simulink model "B_ctrb"  (R2015a)
settings: Solver=ode45  StartTime=0.0  StopTime=50  RelTol=1e-3
values from neighbouring files (symbols this model uses):
  A1 = [-0.125 0 0;1 0 0;0 1 0]    [A_tftf.m]
  B1 = [1;0;0]    [A_tftf.m]
  C1 = [0 -0.0883 -0.0044]    [A_tftf.m]
  D1 = 0    [A_tftf.m]
  K = lqr(a,b,Q,R)    [A_tftf.m]
libraries: simulink x3
settings Model: Creator=HomeTown  LastModifiedBy=HomeTown

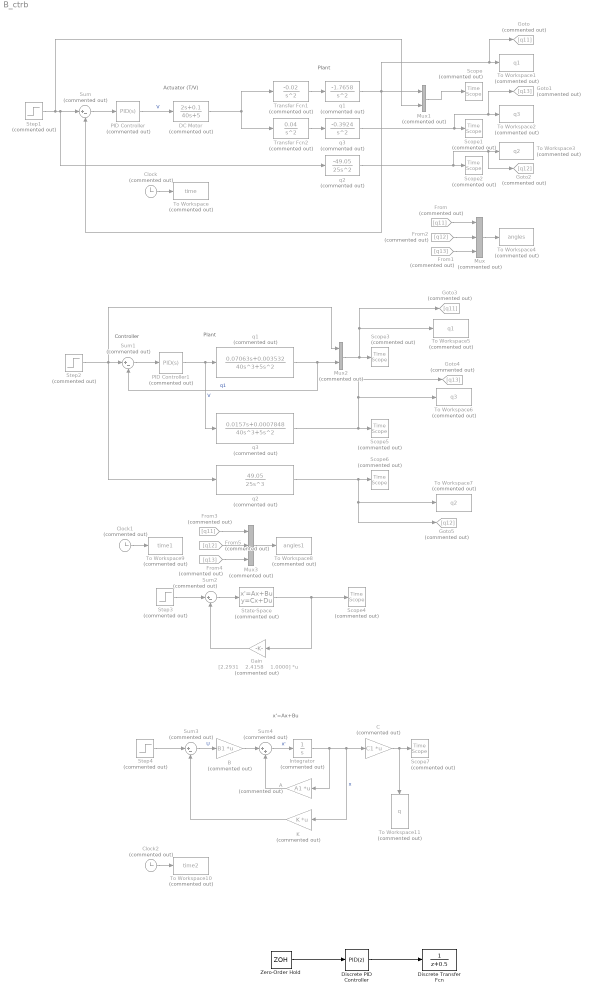
== system B_ctrb ==
  note: x'=Ax+Bu
  note: Controller
  note: Plant
  note: Plant
  note: Actuator (T/V)
  A : Gain  Commented=on  Gain=A1  Multiplication=Matrix(K*u)
  B : Gain  Commented=on  Gain=B1  Multiplication=Matrix(K*u)
  C : Gain  Commented=on  Gain=C1  Multiplication=Matrix(K*u)
  Clock : Clock  Commented=on
  Clock1 : Clock  Commented=on
  Clock2 : Clock  Commented=on
  DC Motor : TransferFcn  Commented=on  Numerator=[2 0.1]  Denominator=[40 5]
  Discrete Transfer Fcn : DiscreteTransferFcn
  Discrete PID Controller : simulink/Continuous/PID Controller  Controller=PID  TimeDomain=Discrete-time  SampleTime=1  IntegratorMethod=Forward Euler  FilterMethod=Forward Euler  Form=Parallel  UseFilter=on  ControllerParametersSource=internal  P=21.1  I=26  D=0  N=100  InitialConditionSource=internal  InitialConditionForIntegrator=0  InitialConditionForFilter=0  ExternalReset=none  LimitOutput=off  UpperSaturationLimit=inf  LowerSaturationLimit=-inf  LinearizeAsGain=off  AntiWindupMode=none  Kb=1  TrackingMode=off  Kt=1  PParamMin=[]  PParamMax=[]  IParamMin=[]  IParamMax=[]  DParamMin=[]  DParamMax=[]  NParamMin=[]  NParamMax=[]  KbParamMin=[]  KbParamMax=[]  KtParamMin=[]  KtParamMax=[]  POutMin=[]  POutMax=[]  IOutMin=[]  IOutMax=[]  DOutMin=[]  DOutMax=[]  NOutMin=[]  NOutMax=[]  KbOutMin=[]  KbOutMax=[]  KtOutMin=[]  KtOutMax=[]  IntegratorOutMin=[]  IntegratorOutMax=[]  FilterOutMin=[]  FilterOutMax=[]  SumOutMin=[]  SumOutMax=[]  SumI1OutMin=[]  SumI1OutMax=[]  SumI2OutMin=[]  SumI2OutMax=[]  SumI3OutMin=[]  SumI3OutMax=[]  SumDOutMin=[]  SumDOutMax=[]  SaturationOutMin=[]  SaturationOutMax=[]  IntegratorContinuousStateAttributes=''  IntegratorStateMustResolveToSignalObject=off  IntegratorRTWStateStorageClass=Auto  FilterContinuousStateAttributes=''  FilterStateMustResolveToSignalObject=off  FilterRTWStateStorageClass=Auto  DifferentiatorICPrevScaledInput=0  DifferentiatorOutMin=[]  DifferentiatorOutMax=[]
  From : From  Commented=on  GotoTag=q11
  From1 : From  Commented=on  GotoTag=q13
  From2 : From  Commented=on  GotoTag=q12
  From3 : From  Commented=on  GotoTag=q11
  From4 : From  Commented=on  GotoTag=q13
  From5 : From  Commented=on  GotoTag=q12
  Gain : Gain  Commented=on  Gain="[2.2931    2.4158    1.0000]"  Multiplication=Matrix(K*u)
  Goto : Goto  Commented=on  GotoTag=q11
  Goto1 : Goto  Commented=on  GotoTag=q13
  Goto2 : Goto  Commented=on  GotoTag=q12
  Goto3 : Goto  Commented=on  GotoTag=q11
  Goto4 : Goto  Commented=on  GotoTag=q13
  Goto5 : Goto  Commented=on  GotoTag=q12
  Integrator : Integrator  Commented=on
  K : Gain  Commented=on  Gain=K  Multiplication=Matrix(K*u)
  Mux : Mux  Commented=on  Inputs=3
  Mux1 : Mux  Commented=on  Inputs=2
  Mux2 : Mux  Commented=on  Inputs=2
  Mux3 : Mux  Commented=on  Inputs=3
  PID Controller : simulink/Continuous/PID Controller  Commented=on  Controller=PID  TimeDomain=Continuous-time  SampleTime=-1  IntegratorMethod=Forward Euler  FilterMethod=Forward Euler  Form=Parallel  UseFilter=on  ControllerParametersSource=internal  P=150000  I=11111  D=11  N=100  InitialConditionSource=internal  InitialConditionForIntegrator=0  InitialConditionForFilter=0  ExternalReset=none  LimitOutput=off  UpperSaturationLimit=inf  LowerSaturationLimit=-inf  LinearizeAsGain=on  AntiWindupMode=none  Kb=1  TrackingMode=off  Kt=1  PParamMin=[]  PParamMax=[]  IParamMin=[]  IParamMax=[]  DParamMin=[]  DParamMax=[]  NParamMin=[]  NParamMax=[]  KbParamMin=[]  KbParamMax=[]  KtParamMin=[]  KtParamMax=[]  POutMin=[]  POutMax=[]  IOutMin=[]  IOutMax=[]  DOutMin=[]  DOutMax=[]  NOutMin=[]  NOutMax=[]  KbOutMin=[]  KbOutMax=[]  KtOutMin=[]  KtOutMax=[]  IntegratorOutMin=[]  IntegratorOutMax=[]  FilterOutMin=[]  FilterOutMax=[]  SumOutMin=[]  SumOutMax=[]  SumI1OutMin=[]  SumI1OutMax=[]  SumI2OutMin=[]  SumI2OutMax=[]  SumI3OutMin=[]  SumI3OutMax=[]  SumDOutMin=[]  SumDOutMax=[]  SaturationOutMin=[]  SaturationOutMax=[]  IntegratorContinuousStateAttributes=''  IntegratorStateMustResolveToSignalObject=off  IntegratorRTWStateStorageClass=Auto  FilterContinuousStateAttributes=''  FilterStateMustResolveToSignalObject=off  FilterRTWStateStorageClass=Auto  DifferentiatorICPrevScaledInput=0  DifferentiatorOutMin=[]  DifferentiatorOutMax=[]
  PID Controller1 : simulink/Continuous/PID Controller  Commented=on  Controller=PID  TimeDomain=Continuous-time  SampleTime=-1  IntegratorMethod=Forward Euler  FilterMethod=Forward Euler  Form=Parallel  UseFilter=on  ControllerParametersSource=internal  P=350.723372354877  I=32.5997950441357  D=893.162577651587  N=8.93309035821885  InitialConditionSource=internal  InitialConditionForIntegrator=0  InitialConditionForFilter=0  ExternalReset=none  LimitOutput=off  UpperSaturationLimit=inf  LowerSaturationLimit=-inf  LinearizeAsGain=on  AntiWindupMode=none  Kb=1  TrackingMode=off  Kt=1  PParamMin=[]  PParamMax=[]  IParamMin=[]  IParamMax=[]  DParamMin=[]  DParamMax=[]  NParamMin=[]  NParamMax=[]  KbParamMin=[]  KbParamMax=[]  KtParamMin=[]  KtParamMax=[]  POutMin=[]  POutMax=[]  IOutMin=[]  IOutMax=[]  DOutMin=[]  DOutMax=[]  NOutMin=[]  NOutMax=[]  KbOutMin=[]  KbOutMax=[]  KtOutMin=[]  KtOutMax=[]  IntegratorOutMin=[]  IntegratorOutMax=[]  FilterOutMin=[]  FilterOutMax=[]  SumOutMin=[]  SumOutMax=[]  SumI1OutMin=[]  SumI1OutMax=[]  SumI2OutMin=[]  SumI2OutMax=[]  SumI3OutMin=[]  SumI3OutMax=[]  SumDOutMin=[]  SumDOutMax=[]  SaturationOutMin=[]  SaturationOutMax=[]  IntegratorContinuousStateAttributes=''  IntegratorStateMustResolveToSignalObject=off  IntegratorRTWStateStorageClass=Auto  FilterContinuousStateAttributes=''  FilterStateMustResolveToSignalObject=off  FilterRTWStateStorageClass=Auto  DifferentiatorICPrevScaledInput=0  DifferentiatorOutMin=[]  DifferentiatorOutMax=[]
  Scope{,1..7} (8 alike) : TimeScope  Commented=on
  State-Space : StateSpace  Commented=on  A=A1  B=B1  C=C1  D=D1  X0=0
  Step1 : Step  Commented=on  SampleTime=0
  Step2 : Step  Commented=on  SampleTime=0
  Step3 : Step  Commented=on  After=0  SampleTime=0
  Step4 : Step  Commented=on  SampleTime=0
  Sum{,1..3} (4 alike) : Sum  Commented=on  Inputs=|+-
  Sum4 : Sum  Commented=on  Inputs=|++
  To Workspace : ToWorkspace  Commented=on  VariableName=time  SampleTime=-1
  To Workspace1 : ToWorkspace  Commented=on  VariableName=q1  SampleTime=-1
  To Workspace10 : ToWorkspace  Commented=on  VariableName=time2  SampleTime=-1
  To Workspace11 : ToWorkspace  Commented=on  VariableName=q  SampleTime=-1
  To Workspace2 : ToWorkspace  Commented=on  VariableName=q3  SampleTime=-1
  To Workspace3 : ToWorkspace  Commented=on  VariableName=q2  SampleTime=-1
  To Workspace4 : ToWorkspace  Commented=on  VariableName=angles  SampleTime=-1
  To Workspace5 : ToWorkspace  Commented=on  VariableName=q1  SampleTime=-1
  To Workspace6 : ToWorkspace  Commented=on  VariableName=q3  SampleTime=-1
  To Workspace7 : ToWorkspace  Commented=on  VariableName=q2  SampleTime=-1
  To Workspace8 : ToWorkspace  Commented=on  VariableName=angles1  SampleTime=-1
  To Workspace9 : ToWorkspace  Commented=on  VariableName=time1  SampleTime=-1
  Transfer Fcn1 : TransferFcn  Commented=on  Numerator=[-0.02]  Denominator=[1 0 0]
  Transfer Fcn2 : TransferFcn  Commented=on  Numerator=[0.04]  Denominator=[1 0 0]
  Zero-Order Hold : ZeroOrderHold
  q1 : TransferFcn  Commented=on  Numerator=[-1.7658]  Denominator=[1 0 0]
  "q1  " : TransferFcn  Commented=on  Numerator=[0.07063 0.003532]  Denominator=[40 5 0 0]
  q2 : TransferFcn  Commented=on  Numerator=[-49.05]  Denominator=[25 0 0]
  "q2 " : TransferFcn  Commented=on  Numerator=[49.05]  Denominator=[25 0 0 0]
  q3 : TransferFcn  Commented=on  Numerator=[-0.3924]  Denominator=[1 0 0]
  "q3 " : TransferFcn  Commented=on  Numerator=[0.0157 0.0007848]  Denominator=[40 5 0 0]
  wires:
  Step1/1 -> Mux1/2, q2/1, Sum/1
  q1/1 -> Sum/2, Goto/1, To Workspace1/1, Mux1/1
  Transfer Fcn1/1 -> q1/1
  Clock/1 -> To Workspace/1
  q3/1 -> Goto1/1, To Workspace2/1, Scope1/1
  Transfer Fcn2/1 -> q3/1
  DC Motor/1 -> Transfer Fcn2/1, Transfer Fcn1/1
  q2/1 -> Goto2/1, To Workspace3/1, Scope2/1
  Mux/1 -> To Workspace4/1
  From/1 -> Mux/1
  From1/1 -> Mux/3
  From2/1 -> Mux/2
  Sum/1 -> PID Controller/1
  PID Controller/1 -> DC Motor/1  "V"
  Mux1/1 -> Scope/1
  Step2/1 -> Mux2/1, "q2 "/1, Sum1/1
  Sum1/1 -> PID Controller1/1
  Mux2/1 -> Goto3/1, To Workspace5/1, Scope3/1
  PID Controller1/1 -> "q3 "/1, "q1  "/1  "V"
  "q1  "/1 -> Sum1/2, Mux2/2  "q1"
  Mux3/1 -> To Workspace8/1
  From3/1 -> Mux3/1
  From4/1 -> Mux3/3
  From5/1 -> Mux3/2
  "q3 "/1 -> Goto4/1, To Workspace6/1, Scope5/1
  "q2 "/1 -> Goto5/1, To Workspace7/1, Scope6/1
  Clock1/1 -> To Workspace9/1
  Sum2/1 -> State-Space/1
  Gain/1 -> Sum2/2
  State-Space/1 -> Gain/1, Scope4/1
  Step3/1 -> Sum2/1
  B/1 -> Sum4/1
  Sum4/1 -> Integrator/1  "x'"
  A/1 -> Sum4/2
  Integrator/1 -> K/1, C/1, A/1  "x"
  C/1 -> Scope7/1, To Workspace11/1
  Step4/1 -> Sum3/1
  K/1 -> Sum3/2
  Sum3/1 -> B/1  "U"
  Clock2/1 -> To Workspace10/1
  Discrete PID Controller/1 -> Discrete Transfer Fcn/1
  Zero-Order Hold/1 -> Discrete PID Controller/1
